simulink model "StateSpace"  (R2021a)
settings: Solver=VariableStepAuto  StartTime=0.0  StopTime=Tfinal  RelTol=1e-3
values from neighbouring files (symbols this model uses):
  K = place(sysD.A,sysD.B,pd)    [Project.m]    (also in SysID.m = x(3); bodeFit.m = x(3))
  sysD = c2d(sys,Ts)    [Project.m]
  Ts = 500e-6*4    (= 0.002)    [Project.m]    (also in ProjectComplementaryFilter.m = 0.00144; Test3D2.m = 0.01)
  Vmax = 12    [Project.m]
  X0 = [deg2rad(attemptedAngle); 0; 0]    [Project.m]
settings Model: Creator=jrs32  LastModifiedBy=jrs32
settings SolverCC: AlgebraicLoopSolver=TrustRegion
settings DebuggingCC: SFMachineParentedDataDiag=warning

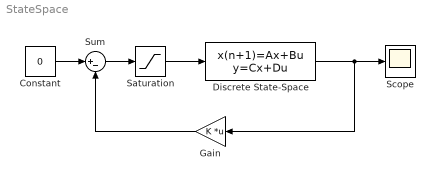
== system StateSpace ==
  Constant : Constant  Value=0
  Discrete State-Space : DiscreteStateSpace  A=sysD.A  B=sysD.B  C=sysD.C  D=sysD.D  InitialCondition=X0  SampleTime=Ts
  Gain : Gain  Gain=K  Multiplication=Matrix(K*u)
  Saturation : Saturate  UpperLimit=Vmax  LowerLimit=-Vmax
  Scope : Scope
  Sum : Sum  Inputs=|+-
  wires:
  Sum/1 -> Saturation/1
  Discrete State-Space/1 -> Scope/1, Gain/1
  Gain/1 -> Sum/2
  Constant/1 -> Sum/1
  Saturation/1 -> Discrete State-Space/1
